simulink model "parallel_8_min_cost_function"  (R2022a)
settings: Solver=FixedStepDiscrete  StartTime=0.0  StopTime=10.0  RelTol=1e-3
undefined symbols (not defined in the file or in its folder): f_c
libraries: hdlsllib x10
settings Model: DataTypeOverride=Off  Creator=Andre Merx  LastModifiedBy=Andre Merx
settings SolverCC: AlgebraicLoopSolver=TrustRegion
settings DataIOCC: LimitDataPoints=on  SaveOutput=off  SaveTime=off
settings OptimizationCC: BlockReduction=off  ConditionallyExecuteInputs=off  DefaultParameterBehavior=Inlined  LifeSpan=inf
settings DebuggingCC: AlgebraicLoopMsg=error  SingleTaskRateTransMsg=error  UnconnectedInputMsg=warning  UnconnectedOutputMsg=warning  UnconnectedLineMsg=warning  AllowSymbolicDim=off  StrictBusMsg=ErrorOnBusTreatedAsVector  SFUnexpectedBacktrackingDiag=warning  SFNoUnconditionalDefaultTransitionDiag=warning  SFExecutionAtInitializationDiag=none  SFMachineParentedDataDiag=warning  ArithmeticOperatorsInVariantConditions=warning
settings HardwareCC: ProdBitPerPointer=32  ProdBitPerSizeT=32  ProdBitPerPtrDiffT=32  ProdLargestAtomicFloat=None  ProdIntDivRoundTo=Undefined  ProdEndianess=Unspecified  ProdWordSize=32  ProdHWDeviceType=ASIC/FPGA->ASIC/FPGA  ProdEqTarget=off
settings SFSimCC: SimUseLocalCustomCode=off  CustomCodeUndefinedFunction=UseInterfaceOnly
settings RTWCC: RTWUseLocalCustomCode=off
settings CodeAppCC: StateflowObjectComments=on
settings GRTTargetCC: TargetLangStandard=C89/C90 (ANSI)
settings ConfigComp: CovScope=ReferencedModels  CovMetricSettings=dw  CovSaveCumulativeToWorkspaceVar=on  CovSaveSingleToWorkspaceVar=on  CovExternalEMLEnable=off  CovSFcnEnable=off

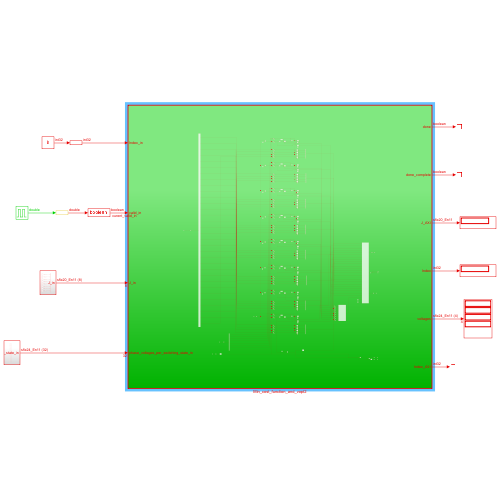
[thumbnail: Simulink's stored preview of the top-level diagram]
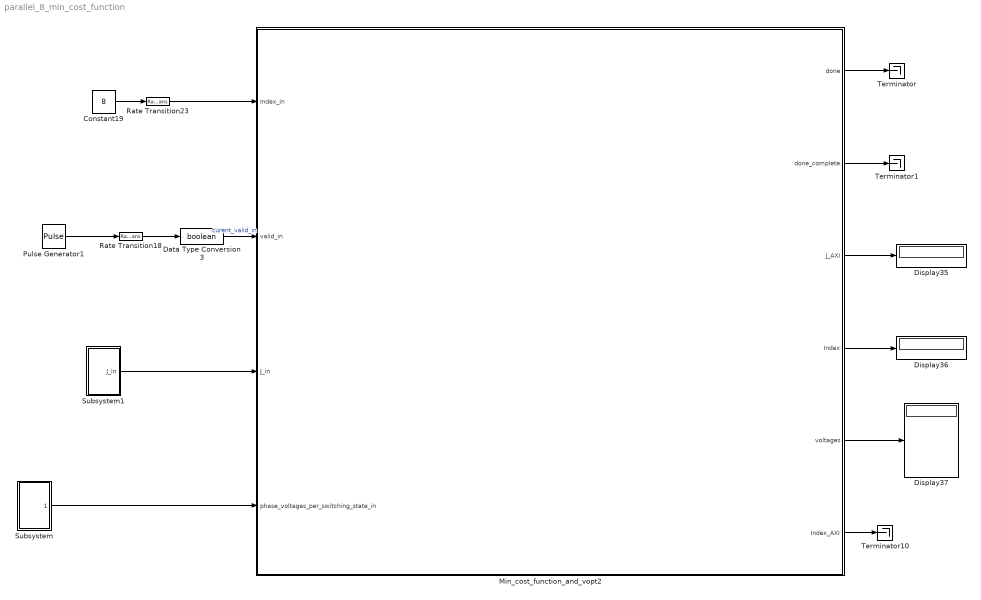
== system parallel_8_min_cost_function ==
  Constant19 : Constant  Value=8  OutDataTypeStr=int32  SampleTime=-1
  Data Type Conversion3 : DataTypeConversion  OutDataTypeStr=boolean  SaturateOnIntegerOverflow=off  RndMeth=Floor
  Display35 : Display
  Display36 : Display
  Display37 : Display
  Min_cost_function_and_vopt2 : Subsystem  TreatAsAtomicUnit=on
  Pulse Generator1 : DiscretePulseGenerator  PulseType=Time based  Period=1/f_c
  Rate Transition18 : RateTransition  OutPortSampleTime=Rt
  Rate Transition23 : RateTransition  OutPortSampleTime=Rt
  Subsystem : Subsystem
  Subsystem1 : Subsystem
  Terminator : Terminator
  Terminator1 : Terminator
  Terminator10 : Terminator
  wires:
  Min_cost_function_and_vopt2/5(voltages) -> Display37/1
  Min_cost_function_and_vopt2/4(Index) -> Display36/1
  Min_cost_function_and_vopt2/3(J_AXI) -> Display35/1
  Min_cost_function_and_vopt2/1(done) -> Terminator/1
  Subsystem/1(phase_voltages_per_switching_state_in) -> Min_cost_function_and_vopt2/4(phase_voltages_per_switching_state_in)
  Subsystem1/1(J_in) -> Min_cost_function_and_vopt2/3(J_in)
  Min_cost_function_and_vopt2/2(done_complete) -> Terminator1/1
  Min_cost_function_and_vopt2/6(Index_AXI) -> Terminator10/1
  Constant19/1 -> Rate Transition23/1
  Rate Transition23/1 -> Min_cost_function_and_vopt2/1(Index_in)
  Data Type Conversion3/1 -> Min_cost_function_and_vopt2/2(valid_in)  "curent_valid_in"
  Pulse Generator1/1 -> Rate Transition18/1
  Rate Transition18/1 -> Data Type Conversion3/1

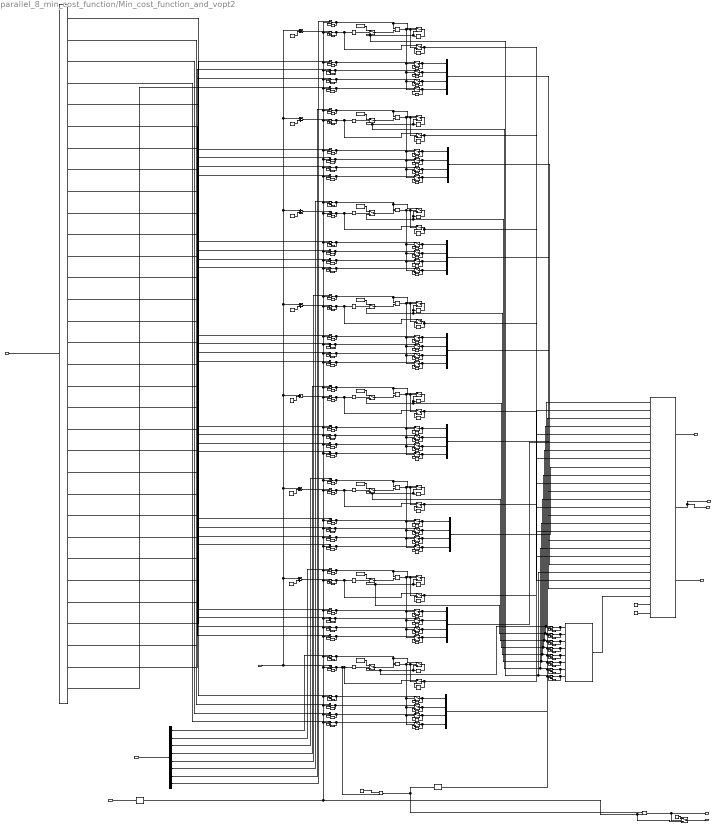
== system parallel_8_min_cost_function/Min_cost_function_and_vopt2 ==
  Index_in : Inport
  valid_in : Inport  Port=2
  J_in : Inport  Port=3
  phase_voltages_per_switching_state_in : Inport  Port=4
  Add{,1..6} (7 alike) : Sum
  Compare To Constant : hdlsllib/Logic and Bit Operations/Compare To Constant  relop=<=  const=1  OutDataTypeStr=boolean
      settings: SourceProductBaseCode=SL
  Compare To Constant1 : hdlsllib/Logic and Bit Operations/Compare To Constant  relop=<=  const=9  OutDataTypeStr=boolean
      settings: SourceProductBaseCode=SL
  Compare To Constant2 : hdlsllib/Logic and Bit Operations/Compare To Constant  relop=<=  const=17  OutDataTypeStr=boolean
      settings: SourceProductBaseCode=SL
  Compare To Constant3 : hdlsllib/Logic and Bit Operations/Compare To Constant  relop=<=  const=25  OutDataTypeStr=boolean
      settings: SourceProductBaseCode=SL
  Compare To Constant4 : hdlsllib/Logic and Bit Operations/Compare To Constant  relop=<=  const=33  OutDataTypeStr=boolean
      settings: SourceProductBaseCode=SL
  Compare To Constant5 : hdlsllib/Logic and Bit Operations/Compare To Constant  relop=<=  const=41  OutDataTypeStr=boolean
      settings: SourceProductBaseCode=SL
  Compare To Constant6 : hdlsllib/Logic and Bit Operations/Compare To Constant  relop=<=  const=49  OutDataTypeStr=boolean
      settings: SourceProductBaseCode=SL
  Compare To Constant7 : hdlsllib/Logic and Bit Operations/Compare To Constant  relop=<=  const=57  OutDataTypeStr=boolean
      settings: SourceProductBaseCode=SL
  Constant{,3..9} (8 alike) : Constant  Value=250  OutDataTypeStr=fixdt(1,20,11)  SampleTime=-1
  Constant1 : Constant  Value=8  OutDataTypeStr=int32  SampleTime=-1
  Constant18 : Constant  Value=8  OutDataTypeStr=int32  SampleTime=-1
  Constant19 : Constant  Value=16  OutDataTypeStr=int32  SampleTime=-1
  Constant2 : Constant  Value=0  OutDataTypeStr=boolean  SampleTime=-1
  Constant20 : Constant  Value=24  OutDataTypeStr=int32  SampleTime=-1
  Constant21 : Constant  Value=32  OutDataTypeStr=int32  SampleTime=-1
  Constant22 : Constant  Value=40  OutDataTypeStr=int32  SampleTime=-1
  Constant23 : Constant  Value=48  OutDataTypeStr=int32  SampleTime=-1
  Constant24 : Constant  Value=56  OutDataTypeStr=int32  SampleTime=-1
  Constant33 : Constant  Value=0  OutDataTypeStr=fixdt(1,20,11)  SampleTime=-1
  Constant34 : Constant  Value=[0;0;0;0]  OutDataTypeStr=fixdt(1,24,11)  SampleTime=-1
  Delay{,1..5,17..22,25..26,34..43,49..50,58..67,72..73,81..90,95..96,104..113,118..119,127..136,141..142,150..159,164..165,173..182,371..378} (104 alike) : Delay  DelayLength=1
  Demux : Demux  Outputs=8
  Demux1 : Demux  Outputs=32
  Detect Rise Positive : hdlsllib/Logic and Bit Operations/Detect Rise Positive  vinit=0  OutDataTypeStr=boolean
      settings: SourceProductBaseCode=SL
  Detect Rise Positive1 : hdlsllib/Logic and Bit Operations/Detect Rise Positive  vinit=0  OutDataTypeStr=boolean
      settings: SourceProductBaseCode=SL
  Logical Operator : Logic  AllPortsSameDT=off  OutDataTypeStr=boolean
  MATLAB Function : MATLAB Function  TreatAsAtomicUnit=on
  MinMax : MinMax  Inputs=8
  Mux{,1..7} (8 alike) : Mux
  Relational Operator{,2..8} (8 alike) : RelationalOperator  Operator=<=  OutDataTypeStr=boolean  RndMeth=Simplest  InputSameDT=off
  Relational Operator1 : RelationalOperator  Operator===  OutDataTypeStr=boolean  RndMeth=Simplest  InputSameDT=off
  Switch{,1,8..9,20..21,27..28,34..35,41..42,48..49,55..56} (16 alike) : Switch  Criteria=u2 > Threshold  OutDataTypeStr=fixdt(1,20,11)  SaturateOnIntegerOverflow=off  InputSameDT=off
  Switch{2,10,15,22,29,36,43,50} (8 alike) : Switch  Criteria=u2 > Threshold  OutDataTypeStr=int32  SaturateOnIntegerOverflow=off  InputSameDT=off
  Switch{3..6,11..14,16..19,23..26,30..33,37..40,44..47,51..54} (32 alike) : Switch  Criteria=u2 > Threshold  OutDataTypeStr=fixdt(1,24,11)  SaturateOnIntegerOverflow=off  InputSameDT=off
  Switch7 : Switch  Criteria=u2 > Threshold  SaturateOnIntegerOverflow=off  InputSameDT=off
  Switch_on{1,4,7,10,14,17,20,23,26,29,32,35,38,41,44,47,98..105} (24 alike) : Switch  Threshold=1  OutDataTypeStr=Inherit: Inherit via back propagation  RndMeth=Simplest  SaturateOnIntegerOverflow=off  InputSameDT=off
  Switch_on{2..3,5..6,8..9,11..12,15..16,18..19,21..22,24..25,27..28,30..31,33..34,36..37,39..40,42..43,45..46,48..49} (32 alike) : Switch  Threshold=1  OutDataTypeStr=fixdt(1,24,11)  RndMeth=Simplest  SaturateOnIntegerOverflow=off  InputSameDT=off
      Switch_on49 settings: LockScale=on
  done : Outport
  done_complete : Outport  Port=2
  J_AXI : Outport  Port=3
  Index : Outport  Port=4
  voltages : Outport  Port=5
  Index_AXI : Outport  Port=6
  wires:
  Demux/1 -> Switch_on4/1  "End_Cycle"
  Demux1/1 -> Switch_on2/1  "End_Cycle"
  Demux1/2 -> Switch_on3/1  "End_Cycle"
  Switch5/1 -> Mux/3, Delay4/1
  Delay3/1 -> Switch4/3
  Relational Operator/1 -> Switch5/2, Switch6/2, Switch4/2, Switch3/2, Switch2/2, Switch1/2
  Compare To Constant/1 -> Switch/2
  Switch1/1 -> Delay/1
  Switch6/1 -> Delay5/1, Mux/4
  Delay4/1 -> Switch5/3
  Switch4/1 -> Mux/2, Delay3/1
  Switch/1 -> Relational Operator/2
  Delay1/1 -> Switch2/3
  Delay5/1 -> Switch6/3
  Switch3/1 -> Mux/1, Delay2/1
  Delay2/1 -> Switch3/3
  Constant/1 -> Switch/1
  Switch_on4/1 -> Relational Operator/1, Switch1/1, Delay17/1
  Switch_on1/1 -> Delay18/1, Relational Operator1/2, Switch2/1, Compare To Constant/1
  Switch_on2/1 -> Delay19/1, Switch3/1
  Switch_on3/1 -> Delay20/1, Switch4/1
  Switch_on5/1 -> Switch5/1, Delay21/1
  Switch_on6/1 -> Switch6/1, Delay22/1
  valid_in/1 -> Detect Rise Positive/1  "End_Cycle"
  Delay17/1 -> Switch_on4/3
  Delay18/1 -> Switch_on1/3
  Delay19/1 -> Switch_on2/3
  Delay20/1 -> Switch_on3/3
  Delay21/1 -> Switch_on5/3
  Delay22/1 -> Switch_on6/3
  Constant1/1 -> Relational Operator1/1
  Constant2/1 -> Switch7/1
  Demux1/3 -> Switch_on5/1  "End_Cycle"
  Demux1/4 -> Switch_on6/1  "End_Cycle"
  Demux/2 -> Switch_on10/1  "End_Cycle"
  Delay34/1 -> Switch_on10/3
  Switch8/1 -> Relational Operator2/2
  Switch_on8/1 -> Delay36/1, Switch11/1
  Demux1/6 -> Switch_on9/1  "End_Cycle"
  Delay26/1 -> Switch10/3
  Add/1 -> Switch_on7/1
  Delay36/1 -> Switch_on8/3
  Delay39/1 -> Switch_on11/3
  Switch_on7/1 -> Delay35/1, Switch10/1, Compare To Constant1/1
  Compare To Constant1/1 -> Switch8/2
  Switch_on9/1 -> Delay38/1, Switch12/1
  Delay40/1 -> Switch_on12/3
  Delay35/1 -> Switch_on7/3
  Switch_on11/1 -> Switch13/1, Delay39/1
  Delay43/1 -> Switch14/3
  Switch_on12/1 -> Switch14/1, Delay40/1
  Delay37/1 -> Switch11/3
  Relational Operator2/1 -> Switch13/2, Switch14/2, Switch12/2, Switch11/2, Switch10/2, Switch9/2
  Switch9/1 -> Delay25/1
  Delay42/1 -> Switch13/3
  Demux1/5 -> Switch_on8/1  "End_Cycle"
  Demux1/7 -> Switch_on11/1  "End_Cycle"
  Switch_on10/1 -> Relational Operator2/1, Switch9/1, Delay34/1
  Demux1/8 -> Switch_on12/1  "End_Cycle"
  Delay38/1 -> Switch_on9/3
  Constant3/1 -> Switch8/1
  Delay41/1 -> Switch12/3
  Delay61/1 -> Switch16/3
  Switch_on16/1 -> Switch19/1, Delay64/1
  Delay67/1 -> Switch19/3
  Switch_on15/1 -> Switch18/1, Delay63/1
  Delay59/1 -> Switch_on17/3
  Switch_on19/1 -> Delay62/1, Switch17/1
  Delay64/1 -> Switch_on16/3
  Switch_on17/1 -> Delay59/1, Switch15/1, Compare To Constant2/1
  Compare To Constant2/1 -> Switch20/2
  Demux1/10 -> Switch_on19/1  "End_Cycle"
  Delay50/1 -> Switch15/3
  Switch20/1 -> Relational Operator3/2
  Demux/3 -> Switch_on14/1  "End_Cycle"
  Delay65/1 -> Switch17/3
  Switch_on14/1 -> Relational Operator3/1, Switch21/1, Delay58/1
  Switch_on18/1 -> Delay60/1, Switch16/1
  Constant4/1 -> Switch20/1
  Demux1/11 -> Switch_on15/1  "End_Cycle"
  Delay63/1 -> Switch_on15/3
  Delay66/1 -> Switch18/3
  Switch21/1 -> Delay49/1
  Demux1/9 -> Switch_on18/1  "End_Cycle"
  Demux1/12 -> Switch_on16/1  "End_Cycle"
  Add1/1 -> Switch_on17/1
  Delay60/1 -> Switch_on18/3
  Relational Operator3/1 -> Switch18/2, Switch19/2, Switch17/2, Switch16/2, Switch15/2, Switch21/2
  Delay58/1 -> Switch_on14/3
  Delay62/1 -> Switch_on19/3
  Delay84/1 -> Switch23/3
  Switch_on22/1 -> Switch26/1, Delay87/1
  Delay90/1 -> Switch26/3
  Switch_on21/1 -> Switch25/1, Delay86/1
  Delay82/1 -> Switch_on23/3
  Switch_on25/1 -> Delay85/1, Switch24/1
  Delay87/1 -> Switch_on22/3
  Switch_on23/1 -> Delay82/1, Switch22/1, Compare To Constant3/1
  Compare To Constant3/1 -> Switch27/2
  Demux1/14 -> Switch_on25/1  "End_Cycle"
  Delay73/1 -> Switch22/3
  Switch27/1 -> Relational Operator4/2
  Demux/4 -> Switch_on20/1  "End_Cycle"
  Delay88/1 -> Switch24/3
  Switch_on20/1 -> Relational Operator4/1, Switch28/1, Delay81/1
  Switch_on24/1 -> Delay83/1, Switch23/1
  Constant5/1 -> Switch27/1
  Demux1/15 -> Switch_on21/1  "End_Cycle"
  Delay86/1 -> Switch_on21/3
  Delay89/1 -> Switch25/3
  Switch28/1 -> Delay72/1
  Demux1/13 -> Switch_on24/1  "End_Cycle"
  Demux1/16 -> Switch_on22/1  "End_Cycle"
  Add2/1 -> Switch_on23/1
  Delay83/1 -> Switch_on24/3
  Relational Operator4/1 -> Switch25/2, Switch26/2, Switch24/2, Switch23/2, Switch22/2, Switch28/2
  Delay81/1 -> Switch_on20/3
  Delay85/1 -> Switch_on25/3
  Delay107/1 -> Switch30/3
  Switch_on28/1 -> Switch33/1, Delay110/1
  Delay113/1 -> Switch33/3
  Switch_on27/1 -> Switch32/1, Delay109/1
  Delay105/1 -> Switch_on29/3
  Switch_on31/1 -> Delay108/1, Switch31/1
  Delay110/1 -> Switch_on28/3
  Switch_on29/1 -> Delay105/1, Switch29/1, Compare To Constant4/1
  Compare To Constant4/1 -> Switch34/2
  Demux1/18 -> Switch_on31/1  "End_Cycle"
  Delay96/1 -> Switch29/3
  Switch34/1 -> Relational Operator5/2
  Demux/5 -> Switch_on26/1  "End_Cycle"
  Delay111/1 -> Switch31/3
  Switch_on26/1 -> Relational Operator5/1, Switch35/1, Delay104/1
  Switch_on30/1 -> Delay106/1, Switch30/1
  Constant6/1 -> Switch34/1
  Demux1/19 -> Switch_on27/1  "End_Cycle"
  Delay109/1 -> Switch_on27/3
  Delay112/1 -> Switch32/3
  Switch35/1 -> Delay95/1
  Demux1/17 -> Switch_on30/1  "End_Cycle"
  Demux1/20 -> Switch_on28/1  "End_Cycle"
  Add3/1 -> Switch_on29/1
  Delay106/1 -> Switch_on30/3
  Relational Operator5/1 -> Switch32/2, Switch33/2, Switch31/2, Switch30/2, Switch29/2, Switch35/2
  Delay104/1 -> Switch_on26/3
  Delay108/1 -> Switch_on31/3
  Delay130/1 -> Switch37/3
  Switch_on34/1 -> Switch40/1, Delay133/1
  Delay136/1 -> Switch40/3
  Switch_on33/1 -> Switch39/1, Delay132/1
  Delay128/1 -> Switch_on35/3
  Switch_on37/1 -> Delay131/1, Switch38/1
  Delay133/1 -> Switch_on34/3
  Switch_on35/1 -> Delay128/1, Switch36/1, Compare To Constant5/1
  Compare To Constant5/1 -> Switch41/2
  Demux1/22 -> Switch_on37/1  "End_Cycle"
  Delay119/1 -> Switch36/3
  Switch41/1 -> Relational Operator6/2
  Demux/6 -> Switch_on32/1  "End_Cycle"
  Delay134/1 -> Switch38/3
  Switch_on32/1 -> Relational Operator6/1, Switch42/1, Delay127/1
  Switch_on36/1 -> Delay129/1, Switch37/1
  Constant7/1 -> Switch41/1
  Demux1/23 -> Switch_on33/1  "End_Cycle"
  Delay132/1 -> Switch_on33/3
  Delay135/1 -> Switch39/3
  Switch42/1 -> Delay118/1
  Demux1/21 -> Switch_on36/1  "End_Cycle"
  Demux1/24 -> Switch_on34/1  "End_Cycle"
  Add4/1 -> Switch_on35/1
  Delay129/1 -> Switch_on36/3
  Relational Operator6/1 -> Switch39/2, Switch40/2, Switch38/2, Switch37/2, Switch36/2, Switch42/2
  Delay127/1 -> Switch_on32/3
  Delay131/1 -> Switch_on37/3
  Delay153/1 -> Switch44/3
  Switch_on40/1 -> Switch47/1, Delay156/1
  Delay159/1 -> Switch47/3
  Switch_on39/1 -> Switch46/1, Delay155/1
  Delay151/1 -> Switch_on41/3
  Switch_on43/1 -> Delay154/1, Switch45/1
  Delay156/1 -> Switch_on40/3
  Switch_on41/1 -> Delay151/1, Switch43/1, Compare To Constant6/1
  Compare To Constant6/1 -> Switch48/2
  Demux1/26 -> Switch_on43/1  "End_Cycle"
  Delay142/1 -> Switch43/3
  Switch48/1 -> Relational Operator7/2
  Delay157/1 -> Switch45/3
  Switch_on38/1 -> Relational Operator7/1, Switch49/1, Delay150/1
  Switch_on42/1 -> Delay152/1, Switch44/1
  Constant8/1 -> Switch48/1
  Demux1/27 -> Switch_on39/1  "End_Cycle"
  Delay155/1 -> Switch_on39/3
  Delay158/1 -> Switch46/3
  Switch49/1 -> Delay141/1
  Demux1/25 -> Switch_on42/1  "End_Cycle"
  Demux1/28 -> Switch_on40/1  "End_Cycle"
  Add5/1 -> Switch_on41/1
  Delay152/1 -> Switch_on42/3
  Relational Operator7/1 -> Switch46/2, Switch47/2, Switch45/2, Switch44/2, Switch43/2, Switch49/2
  Delay150/1 -> Switch_on38/3
  Delay154/1 -> Switch_on43/3
  Delay176/1 -> Switch51/3
  Switch_on46/1 -> Switch54/1, Delay179/1
  Delay182/1 -> Switch54/3
  Switch_on45/1 -> Switch53/1, Delay178/1
  Delay174/1 -> Switch_on47/3
  Switch_on49/1 -> Delay177/1, Switch52/1
  Delay179/1 -> Switch_on46/3
  Switch_on47/1 -> Delay174/1, Switch50/1, Compare To Constant7/1
  Compare To Constant7/1 -> Switch55/2
  Demux1/30 -> Switch_on49/1  "End_Cycle"
  Delay165/1 -> Switch50/3
  Switch55/1 -> Relational Operator8/2
  Demux/8 -> Switch_on44/1  "End_Cycle"
  Delay180/1 -> Switch52/3
  Switch_on44/1 -> Relational Operator8/1, Switch56/1, Delay173/1
  Switch_on48/1 -> Delay175/1, Switch51/1
  Constant9/1 -> Switch55/1
  Demux1/31 -> Switch_on45/1  "End_Cycle"
  Delay178/1 -> Switch_on45/3
  Delay181/1 -> Switch53/3
  Switch56/1 -> Delay164/1
  Demux1/29 -> Switch_on48/1  "End_Cycle"
  Demux1/32 -> Switch_on46/1  "End_Cycle"
  Add6/1 -> Switch_on47/1
  Delay175/1 -> Switch_on48/3
  Relational Operator8/1 -> Switch53/2, Switch54/2, Switch52/2, Switch51/2, Switch50/2, Switch56/2
  Delay173/1 -> Switch_on44/3
  Delay177/1 -> Switch_on49/3
  Detect Rise Positive/1 -> Switch7/3, Logical Operator/2, Switch_on44/2, Switch_on47/2, Switch_on48/2, Switch_on49/2, Switch_on45/2, Switch_on46/2, Switch_on38/2, Switch_on41/2, Switch_on42/2, Switch_on43/2, Switch_on39/2, Switch_on40/2, Switch_on32/2, Switch_on35/2, Switch_on36/2, Switch_on37/2, Switch_on33/2, Switch_on34/2, Switch_on26/2, Switch_on29/2, Switch_on30/2, Switch_on31/2, Switch_on27/2, Switch_on28/2, Switch_on20/2, Switch_on23/2, Switch_on24/2, Switch_on25/2, Switch_on21/2, Switch_on22/2, Switch_on14/2, Switch_on17/2, Switch_on18/2, Switch_on19/2, Switch_on15/2, Switch_on16/2, Switch_on10/2, Switch_on7/2, Switch_on8/2, Switch_on9/2, Switch_on11/2, Switch_on12/2, Switch_on4/2, Switch_on1/2, Switch_on2/2, Switch_on3/2, Switch_on5/2, Switch_on6/2  "End_Cycle"
  Constant18/1 -> Add/2
  Constant19/1 -> Add1/2
  Constant20/1 -> Add2/2
  Constant21/1 -> Add3/2
  Constant22/1 -> Add4/2
  Constant23/1 -> Add5/2
  Constant24/1 -> Add6/2
  Delay371/1 -> Switch_on98/3
  Switch_on98/1 -> Delay371/1, MinMax/1
  Switch_on99/1 -> Delay372/1, MinMax/2
  Delay372/1 -> Switch_on99/3
  Switch_on100/1 -> Delay373/1, MinMax/3
  Delay373/1 -> Switch_on100/3
  Switch_on101/1 -> Delay374/1, MinMax/4
  Delay374/1 -> Switch_on101/3
  Delay376/1 -> Switch_on105/3
  Switch_on102/1 -> Delay377/1, MinMax/7
  Delay377/1 -> Switch_on102/3
  Delay141/1 -> Switch_on102/1, MATLAB Function/19(J_7), Switch48/3, Switch49/3
  Switch_on104/1 -> Delay375/1, MinMax/5
  Delay375/1 -> Switch_on104/3
  Switch_on105/1 -> Delay376/1, MinMax/6
  Switch_on103/1 -> Delay378/1, MinMax/8
  Delay378/1 -> Switch_on103/3
  Relational Operator1/1 -> Detect Rise Positive1/1, Logical Operator/1  "End_Cycle"
  Detect Rise Positive1/1 -> Switch_on98/2, Switch_on99/2, Switch_on100/2, Switch_on101/2, Switch_on104/2, Switch_on105/2, Switch_on102/2, Switch_on103/2  "End_Cycle"
  MinMax/1 -> MATLAB Function/25(min)
  Delay/1 -> Switch_on98/1, MATLAB Function/1(J_1), Switch/3, Switch1/3
  Delay25/1 -> Switch_on99/1, MATLAB Function/4(J_2), Switch8/3, Switch9/3
  Delay49/1 -> Switch_on100/1, MATLAB Function/7(J_3), Switch20/3, Switch21/3
  Delay72/1 -> Switch_on101/1, MATLAB Function/10(J_4), Switch27/3, Switch28/3
  Delay95/1 -> Switch34/3, Switch_on104/1, MATLAB Function/13(J_5), Switch35/3
  Delay118/1 -> Switch41/3, Switch_on105/1, MATLAB Function/16(J_6), Switch42/3
  Delay164/1 -> Switch_on103/1, MATLAB Function/22(J_8), Switch55/3, Switch56/3
  Switch2/1 -> MATLAB Function/2(Index_1), Delay1/1
  Switch10/1 -> MATLAB Function/5(Index_2), Delay26/1
  Switch15/1 -> MATLAB Function/8(Index_3), Delay50/1
  Switch22/1 -> MATLAB Function/11(Index_4), Delay73/1
  Switch29/1 -> MATLAB Function/14(Index_5), Delay96/1
  Switch36/1 -> MATLAB Function/17(Index_6), Delay119/1
  Switch43/1 -> MATLAB Function/20(Index_7), Delay142/1
  Switch50/1 -> MATLAB Function/23(Index_8), Delay165/1
  Switch13/1 -> Mux1/3, Delay42/1
  Switch12/1 -> Mux1/2, Delay41/1
  Switch14/1 -> Mux1/4, Delay43/1
  Switch11/1 -> Mux1/1, Delay37/1
  Switch18/1 -> Mux2/3, Delay66/1
  Switch17/1 -> Mux2/2, Delay65/1
  Switch19/1 -> Mux2/4, Delay67/1
  Switch16/1 -> Mux2/1, Delay61/1
  Switch25/1 -> Delay89/1, Mux3/3
  Switch24/1 -> Mux3/2, Delay88/1
  Switch26/1 -> Mux3/4, Delay90/1
  Switch23/1 -> Mux3/1, Delay84/1
  Switch32/1 -> Mux4/3, Delay112/1
  Switch31/1 -> Mux4/2, Delay111/1
  Switch33/1 -> Mux4/4, Delay113/1
  Switch30/1 -> Delay107/1, Mux4/1
  Switch39/1 -> Mux5/3, Delay135/1
  Switch38/1 -> Delay134/1, Mux5/2
  Switch40/1 -> Mux5/4, Delay136/1
  Switch37/1 -> Mux5/1, Delay130/1
  Switch46/1 -> Mux6/3, Delay158/1
  Switch45/1 -> Mux6/2, Delay157/1
  Switch47/1 -> Mux6/4, Delay159/1
  Switch44/1 -> Mux6/1, Delay153/1
  Switch53/1 -> Mux7/3, Delay181/1
  Switch52/1 -> Mux7/2, Delay180/1
  Switch54/1 -> Mux7/4, Delay182/1
  Switch51/1 -> Mux7/1, Delay176/1
  Mux/1 -> MATLAB Function/3(voltages_1)
  Mux1/1 -> MATLAB Function/6(voltages_2)
  Mux2/1 -> MATLAB Function/9(voltages_3)
  Mux3/1 -> MATLAB Function/12(voltages_4)
  Mux4/1 -> MATLAB Function/15(voltages_5)
  Mux5/1 -> MATLAB Function/18(voltages_6)
  Mux6/1 -> MATLAB Function/21(voltages_7)
  Mux7/1 -> MATLAB Function/24(voltages_8)
  Constant33/1 -> MATLAB Function/26(J_default)
  Constant34/1 -> MATLAB Function/27(voltages_default)
  Demux/7 -> Switch_on38/1  "End_Cycle"
  J_in/1 -> Demux/1  "End_Cycle"
  phase_voltages_per_switching_state_in/1 -> Demux1/1  "End_Cycle"
  Index_in/1 -> Switch_on1/1, Add/1, Add3/1, Add6/1, Add5/1, Add4/1, Add2/1, Add1/1
  Logical Operator/1 -> done_complete/1, Switch7/2
  Switch7/1 -> done/1
  MATLAB Function/3(voltages) -> voltages/1
  MATLAB Function/2(Index) -> Index_AXI/1, Index/1
  MATLAB Function/1(J) -> J_AXI/1

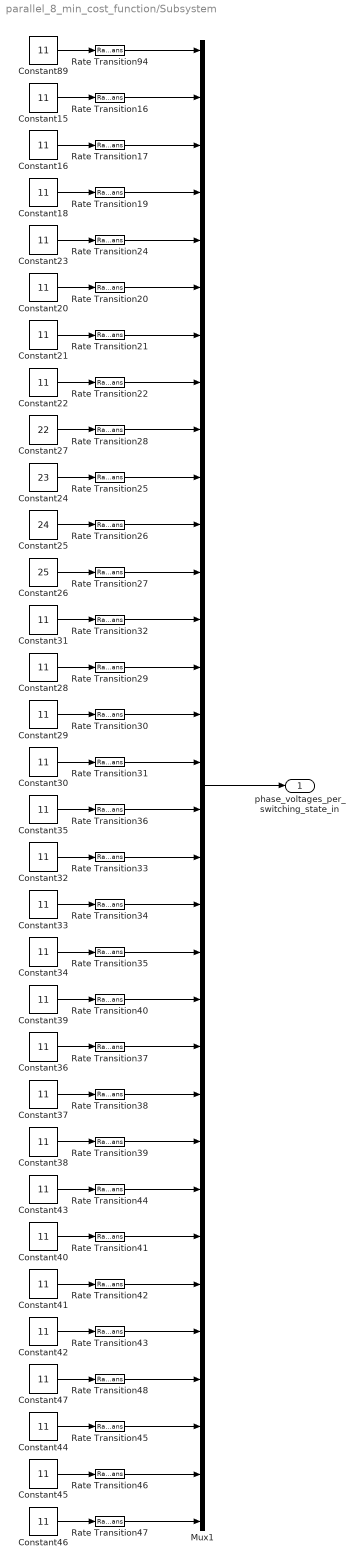
== system parallel_8_min_cost_function/Subsystem ==
  Constant{15..16,18,20..23,28..47,89} (28 alike) : Constant  Value=11  OutDataTypeStr=fixdt(1,24,11)  SampleTime=-1  LockScale=on
  Constant24 : Constant  Value=23  OutDataTypeStr=fixdt(1,24,11)  SampleTime=-1  LockScale=on
  Constant25 : Constant  Value=24  OutDataTypeStr=fixdt(1,24,11)  SampleTime=-1  LockScale=on
  Constant26 : Constant  Value=25  OutDataTypeStr=fixdt(1,24,11)  SampleTime=-1  LockScale=on
  Constant27 : Constant  Value=22  OutDataTypeStr=fixdt(1,24,11)  SampleTime=-1  LockScale=on
  Mux1 : Mux  Inputs=32
  Rate Transition{16..17,19..22,24..48,94} (32 alike) : RateTransition  OutPortSampleTime=Rt
  phase_voltages_per_switching_state_in : Outport  VectorParamsAs1DForOutWhenUnconnected=off
  wires:
  Rate Transition36/1 -> Mux1/17
  Constant35/1 -> Rate Transition36/1
  Constant42/1 -> Rate Transition43/1
  Mux1/1 -> phase_voltages_per_switching_state_in/1
  Constant24/1 -> Rate Transition25/1
  Constant32/1 -> Rate Transition33/1
  Constant18/1 -> Rate Transition19/1
  Rate Transition94/1 -> Mux1/1
  Constant36/1 -> Rate Transition37/1
  Rate Transition34/1 -> Mux1/19
  Constant37/1 -> Rate Transition38/1
  Rate Transition48/1 -> Mux1/29
  Constant43/1 -> Rate Transition44/1
  Constant20/1 -> Rate Transition20/1
  Rate Transition28/1 -> Mux1/9
  Rate Transition16/1 -> Mux1/2
  Constant34/1 -> Rate Transition35/1
  Rate Transition17/1 -> Mux1/3
  Rate Transition39/1 -> Mux1/24
  Constant41/1 -> Rate Transition42/1
  Constant27/1 -> Rate Transition28/1
  Constant47/1 -> Rate Transition48/1
  Constant33/1 -> Rate Transition34/1
  Constant22/1 -> Rate Transition22/1
  Rate Transition32/1 -> Mux1/13
  Constant29/1 -> Rate Transition30/1
  Constant46/1 -> Rate Transition47/1
  Rate Transition24/1 -> Mux1/5
  Rate Transition25/1 -> Mux1/10
  Constant21/1 -> Rate Transition21/1
  Rate Transition45/1 -> Mux1/30
  Constant28/1 -> Rate Transition29/1
  Rate Transition44/1 -> Mux1/25
  Constant30/1 -> Rate Transition31/1
  Rate Transition38/1 -> Mux1/23
  Constant15/1 -> Rate Transition16/1
  Constant31/1 -> Rate Transition32/1
  Constant89/1 -> Rate Transition94/1
  Rate Transition43/1 -> Mux1/28
  Constant44/1 -> Rate Transition45/1
  Constant23/1 -> Rate Transition24/1
  Constant45/1 -> Rate Transition46/1
  Constant16/1 -> Rate Transition17/1
  Constant26/1 -> Rate Transition27/1
  Constant25/1 -> Rate Transition26/1
  Constant40/1 -> Rate Transition41/1
  Rate Transition42/1 -> Mux1/27
  Rate Transition29/1 -> Mux1/14
  Constant38/1 -> Rate Transition39/1
  Rate Transition19/1 -> Mux1/4
  Rate Transition30/1 -> Mux1/15
  Rate Transition21/1 -> Mux1/7
  Rate Transition22/1 -> Mux1/8
  Rate Transition33/1 -> Mux1/18
  Rate Transition20/1 -> Mux1/6
  Rate Transition27/1 -> Mux1/12
  Rate Transition40/1 -> Mux1/21
  Rate Transition46/1 -> Mux1/31
  Rate Transition26/1 -> Mux1/11
  Rate Transition47/1 -> Mux1/32
  Rate Transition35/1 -> Mux1/20
  Rate Transition37/1 -> Mux1/22
  Rate Transition31/1 -> Mux1/16
  Rate Transition41/1 -> Mux1/26
  Constant39/1 -> Rate Transition40/1

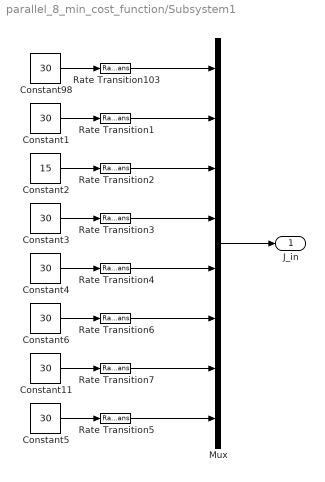
== system parallel_8_min_cost_function/Subsystem1 ==
  Constant{1,3..6,11,98} (7 alike) : Constant  Value=30  OutDataTypeStr=fixdt(1,20,11)  SampleTime=-1
  Constant2 : Constant  Value=15  OutDataTypeStr=fixdt(1,20,11)  SampleTime=-1
  Mux : Mux  Inputs=8
  Rate Transition{1..7,103} (8 alike) : RateTransition  OutPortSampleTime=Rt
  J_in : Outport
  wires:
  Constant1/1 -> Rate Transition1/1
  Rate Transition103/1 -> Mux/1
  Rate Transition5/1 -> Mux/8
  Constant11/1 -> Rate Transition7/1
  Rate Transition4/1 -> Mux/5
  Rate Transition2/1 -> Mux/3
  Constant3/1 -> Rate Transition3/1
  Rate Transition1/1 -> Mux/2
  Constant5/1 -> Rate Transition5/1
  Rate Transition7/1 -> Mux/7
  Constant4/1 -> Rate Transition4/1
  Rate Transition3/1 -> Mux/4
  Constant98/1 -> Rate Transition103/1
  Constant2/1 -> Rate Transition2/1
  Rate Transition6/1 -> Mux/6
  Constant6/1 -> Rate Transition6/1
  Mux/1 -> J_in/1

== matlab function parallel_8_min_cost_function/Min_cost_function_and_vopt2/MATLAB Function ==
  data: J_1 input fixdt(1,20,11); Index_1 input int32; J output fixdt(1,20,11); voltages_1 input fixdt(1,24,11); J_2 input fixdt(1,20,11); Index_2 input int32; voltages_2 input fixdt(1,24,11); J_3 input fixdt(1,20,11); Index_3 input int32; voltages_3 input fixdt(1,24,11); J_4 input fixdt(1,20,11); Index_4 input int32; voltages_4 input fixdt(1,24,11); J_5 input fixdt(1,20,11); Index_5 input int32; voltages_5 input fixdt(1,24,11); J_6 input fixdt(1,20,11); Index_6 input; voltages_6 input fixdt(1,24,11); J_7 input fixdt(1,20,11); Index_7 input int32; voltages_7 input fixdt(1,24,11); J_8 input fixdt(1,20,11); Index_8 input int32; voltages_8 input fixdt(1,24,11); Index output int32; voltages output fixdt(1,24,11); min input fixdt(1,20,11); J_default input fixdt(1,20,11); voltages_default input fixdt(1,24,11)
function [J, Index, voltages] = fcn(J_1, Index_1, voltages_1, J_2, Index_2, voltages_2, J_3, Index_3, voltages_3, J_4, Index_4, voltages_4, J_5, Index_5, voltages_5, J_6, Index_6, voltages_6, ...
                                    J_7, Index_7, voltages_7, J_8, Index_8, voltages_8, min, J_default,voltages_default)



if J_1 == min
    Index = Index_1;
    voltages = voltages_1;
    J = J_1;
elseif J_2 == min
    Index = Index_2;
    voltages = voltages_2;
    J = J_2;
elseif J_3 == min
    Index = Index_3;
    voltages = voltages_3;
    J = J_3;
elseif J_4 == min
    Index = Index_4;
    voltages = voltages_4;
    J = J_4;
elseif J_5 == min
    Index = Index_5;
    voltages = voltages_5;
    J = J_5;
elseif J_6 == min
    Index = Index_6;
    voltages = voltages_6;
    J = J_6;
elseif J_7 == min
    Index = Index_7;
    voltages = voltages_7;
    J = J_7;
elseif J_8 == min
    Index = Index_8;
    voltages = voltages_8;
    J = J_8;
else 
    Index = int32(0);
    J = J_default;
    voltages = voltages_default;
end
